simulink model "I_OSsoftx"  (Simulink 5.0)
settings: Solver=ode45  StartTime=0.0  StopTime=20  RelTol=1e-3
settings Model: LastModifiedBy=User  BlockReductionOpt=off  BooleanDataType=off

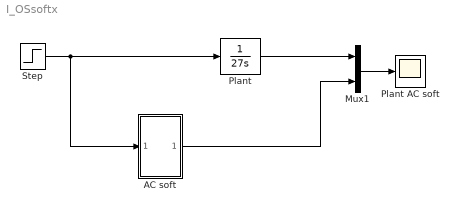
== system I_OSsoftx ==
  AC soft : Subsystem
  Mux1 : Mux  Inputs=2
  Plant : TransferFcn  Denominator=[27 0]
  Plant AC soft : Scope
      settings: YMin=-5e+283  YMax=9e+284
  Step : Step  Time=0.1  SampleTime=0
  wires:
  Step/1 -> Plant/1, AC soft/1(In1)
  Plant/1 -> Mux1/1
  Mux1/1 -> Plant AC soft/1
  AC soft/1(Out1) -> Mux1/2

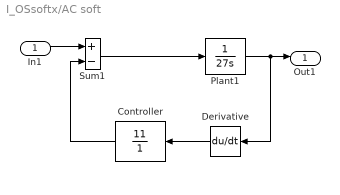
== system I_OSsoftx/AC soft ==
  In1 : Inport
  Controller : TransferFcn  Orientation=left  Numerator=[11]  Denominator=[0 1]
  Derivative : Derivative  Orientation=left
  Plant1 : TransferFcn  Denominator=[27 0]
  Sum1 : Sum  Inputs=+-  SaturateOnIntegerOverflow=on  InputSameDT=on
  Out1 : Outport
  wires:
  Sum1/1 -> Plant1/1
  Plant1/1 -> Derivative/1, Out1/1
  Controller/1 -> Sum1/2
  Derivative/1 -> Controller/1
  In1/1 -> Sum1/1
